simulink subsystem "aqueous_channel"  (R2022b)
settings: Solver=VariableStepAuto  StartTime=0.0  StopTime=10.0  RelTol=1e-3
model mask{C=1, Rc=0, L=L_aq, Rl=0, R=R_aq, UpperSaturationLimit=y_max(1), InitialCondition=0}
  mask prompts: C "Capacitance"; Rc "Series resistance"; L "Inductance"; Rl "Series resistance"; R "Resistance"; UpperSaturationLimit "Simulink:blkprm_prompts:IntegratorUpperSatLim"; InitialCondition "Simulink:blkprm_prompts:IntegratorInitCond"
values from neighbouring files (symbols this model uses):
  dt = 1/samplingRate    (= 0.025)    [plantConstants.m]    (also in sysID.m)
  R = D_est * D_est'    [mpcDesign.m]    (also in stateEst_.m; stateEstimator.m)
undefined symbols (not defined in the file or in its folder): DiscIntNeverNeededParam
libraries: fl_lib x6, nesl_utility x1
settings Model: Creator=khqc  LastModifiedBy=khqc

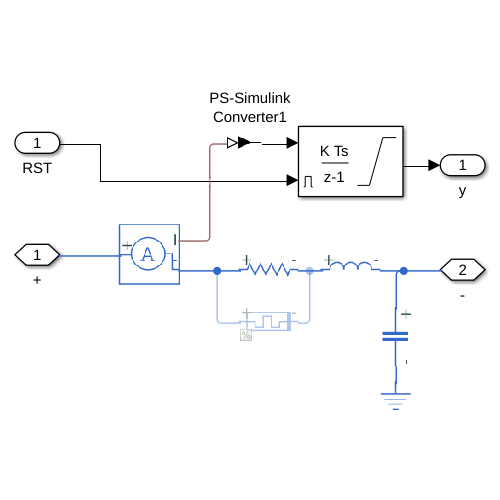
[thumbnail: Simulink's stored preview of the top-level diagram]
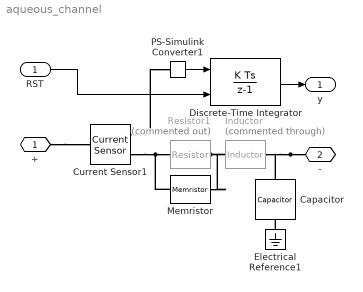
== system aqueous_channel ==
  RST : Inport
  Capacitor : fl_lib/Electrical/Electrical Elements/Capacitor  c=C F  r=Rc Ohm  g=0 1/Ohm  i_specify=off  i_priority=None  i=0 A  i_nominal_specify=off  i_nominal_unit=A  i_nominal_value=1  v_specify=off  v_priority=None  v=0 V  v_nominal_specify=off  v_nominal_unit=V  v_nominal_value=1  vc_specify=off  vc_priority=High  vc=0 V  vc_nominal_specify=off  vc_nominal_unit=V  vc_nominal_value=1
  Current Sensor1 : fl_lib/Electrical/Electrical Sensors/Current Sensor
  Discrete-Time Integrator : DiscreteIntegrator  ExternalReset=level  InitialCondition=InitialCondition  SampleTime=dt  LimitOutput=on  UpperSaturationLimit=UpperSaturationLimit  LowerSaturationLimit=0  ICPrevOutput=DiscIntNeverNeededParam  ICPrevScaledInput=DiscIntNeverNeededParam
  Electrical Reference1 : fl_lib/Electrical/Electrical Elements/Electrical Reference
  Inductor : fl_lib/Electrical/Electrical Elements/Inductor  Commented=through  l=L H  r=Rl Ohm  g=0 1/Ohm  i_specify=off  i_priority=None  i=0 A  i_nominal_specify=off  i_nominal_unit=A  i_nominal_value=1  v_specify=off  v_priority=None  v=0 V  v_nominal_specify=off  v_nominal_unit=V  v_nominal_value=1  i_L_specify=off  i_L_priority=High  i_L=0 A  i_L_nominal_specify=off  i_L_nominal_unit=A  i_L_nominal_value=1
  Memristor : fl_lib/Electrical/Electrical Elements/Memristor  Ra=50*R Ohm  Rb=10*R Ohm  Q0=100 C  x0=0  pwindow=2  i_specify=off  i_priority=None  i=0 A  i_nominal_specify=off  i_nominal_unit=A  i_nominal_value=1  v_specify=off  v_priority=None  v=0 V  v_nominal_specify=off  v_nominal_unit=V  v_nominal_value=1
      settings: InternalSimscapePortConfiguration="{\"Bottom\":[],\"Left\":[{\"id\":\"p\",\"label\":\"+\",\"type\":\"foundation.electrical.electrical\"}],\"Right\":[{\"id\":\"n\",\"label\":\"-\",\"type\":\"foundation.electrical.electrical\"}],\"Top\":[]}"
  PS-Simulink Converter1 : nesl_utility/PS-Simulink Converter  PhysicalDomain=network_engine_domain  SubClassName=ps_output  LeftPortType=input  RightPortType=output  PseudoPeriodic=off  Frequencies=[]  VectorFormat=inherit  Unit=inherit  AffineConversion=off
  Resistor1 : fl_lib/Electrical/Electrical Elements/Resistor  Commented=on  R=R Ohm  i_specify=off  i_priority=None  i=0 A  i_nominal_specify=off  i_nominal_unit=A  i_nominal_value=1  v_specify=off  v_priority=None  v=0 V  v_nominal_specify=off  v_nominal_unit=V  v_nominal_value=1
  + : PMIOPort  Side=Left
  - : PMIOPort  Port=2  Side=Right
  y : Outport
  wires:
  PS-Simulink Converter1/1 -> Discrete-Time Integrator/1
  Discrete-Time Integrator/1 -> y/1
  RST/1 -> Discrete-Time Integrator/2
  connections:
  Memristor/LConn1 -- Resistor1/LConn1 -- Current Sensor1/RConn2
  -/RConn1 -- Capacitor/LConn1 -- Inductor/RConn1
  Inductor/LConn1 -- Memristor/RConn1 -- Resistor1/RConn1
  +/RConn1 -- Current Sensor1/LConn1
  Current Sensor1/RConn1 -- PS-Simulink Converter1/LConn1
  Electrical Reference1/LConn1 -- Capacitor/RConn1
